simulink model "QBot2e_Path_Planning_Motion_Control"  (Simulink 8.9)
settings: Solver=ode1  StartTime=0.0  StopTime=inf  FixedStep=0.01  RelTol=1e-3  EnableMultiTasking=on
values from neighbouring files (symbols this model uses):
  px = wx    [Path_Planning_MAP.m]    (also in Process_MAP.m = coords(:, 1))
  py = wy    [Path_Planning_MAP.m]    (also in Process_MAP.m = coords(:, 2))
undefined symbols (not defined in the file or in its folder): HIL
libraries: quarc_library x8
settings Model: Creator=drmadill  LastModifiedBy=amolki  SimulationMode=external  ExtModeTrigDuration=1
settings SolverCC: PositivePriorityOrder=on
settings OptimizationCC: ExpressionDepthLimit=2147483647  LifeSpan=auto
settings DebuggingCC: SolverPrmCheckMsg=warning
settings RTWCC: SystemTargetFile=quarc_linux_pi_3.tlc  TemplateMakefile=quarc_linux_pi_3_tmf  Description=QUARC Linux Raspberry Pi 3 Target
settings STFCustomTargetCC: TargetLibSuffix=.a  TargetPreCompLibLocation=C:\PROGRA~3\QUARC\lib\2017a\LICFC8~1\release  ConcurrentExecutionCompliant=on  SystemTargetFile=quarc_linux_pi_3.tlc
settings GRTTargetCC: TargetLibSuffix=.a  TargetPreCompLibLocation=C:\PROGRA~3\QUARC\lib\2017a\LICFC8~1\release  ParMdlRefBuildCompliant=off  CompOptLevelCompliant=off  GeneratePreprocessorConditionals=Use local settings  MatFileLogging=off  CPPClassGenCompliant=off  UseToolchainInfoCompliant=off  ExtMode=on  ExtModeMexFile=quarc_comm  ExtModeMexArgs='-w -d /tmp -uri %u'
settings ConfigComp: CovSFcnEnable=off

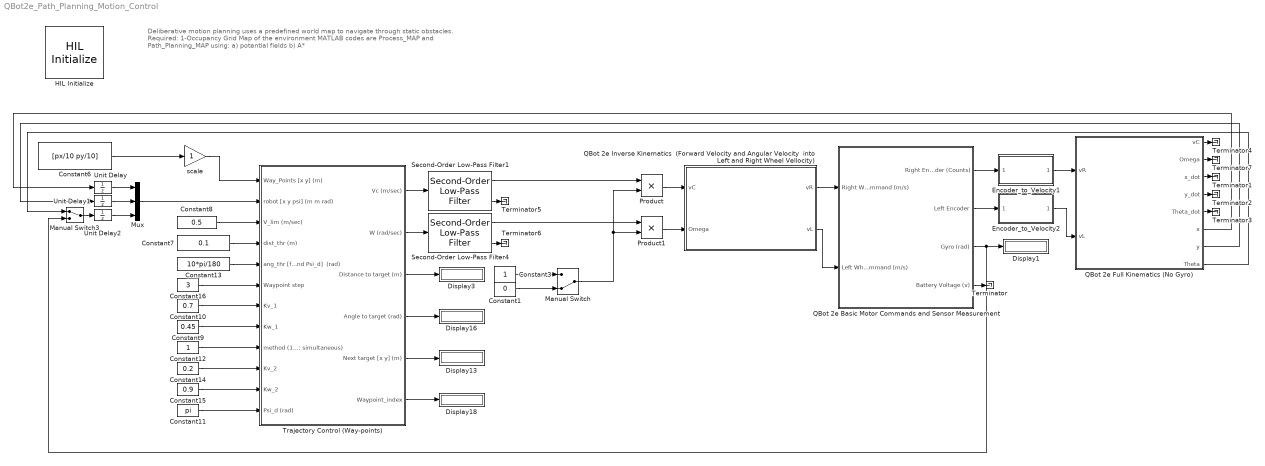
== system QBot2e_Path_Planning_Motion_Control ==
  note: Deliberative motion planning uses a predefined world map to navigate through static obstacles.
      |
      | Required:
      | 1-Occupancy Grid Map of the environment
      | MATLAB codes are Process_MAP and Path_Planning_MAP using:
      | a) potential fields
      | b) A*
  Constant1 : Constant  Value=0
  Constant10 : Constant  Value=0.7
  Constant11 : Constant  Value=pi
  Constant12 : Constant
  Constant13 : Constant  Value=10*pi/180
  Constant14 : Constant  Value=0.2
  Constant15 : Constant  Value=0.9
  Constant16 : Constant  Value=3
  Constant3 : Constant
  Constant6 : Constant  Value=[px/10 py/10]  OutDataTypeStr=double
  Constant7 : Constant  Value=0.1
  Constant8 : Constant  Value=0.5
  Constant9 : Constant  Value=0.45
  Display{1,3,13,16,18} (5 alike) : Display
  Encoder_to_Velocity1 : Subsystem
  Encoder_to_Velocity2 : Subsystem
  HIL Initialize : quarc_library/Data Acquisition/Generic/Configuration/HIL Initialize  Priority=-99  object_name=HIL-1  board_type=qbot2e  board_number=0  board_options=pwm0_en=1;pwm0_pin=12;pwm1_en=1;pwm1_pin=13;  exclusive=off  active=off  hardware_clocks=[]  clock_modes=[]  initial_clock_frequencies=[]  set_clock_params_at_start=off  set_clock_params_at_switch_in=off  set_clock_frequencies_at_start=off  set_clock_frequencies_at_switch_in=off  analog_input_channels=[0:5]  analog_input_configurations=[]  analog_input_maximums=[16.5 3.3 3.3 3.3 3.3 3.3]  analog_input_minimums=[0 0 0 0 0 0]  set_analog_input_params_at_start=off  set_analog_input_params_at_switch_in=off  analog_output_channels=[]  analog_output_maximums=[]  analog_output_minimums=[]  initial_analog_outputs=[]  final_analog_outputs=[]  watchdog_analog_outputs=[]  set_analog_output_params_at_start=off  set_analog_output_params_at_switch_in=off  set_analog_outputs_at_start=off  set_analog_outputs_at_switch_in=off  set_analog_outputs_at_terminate=off  set_analog_outputs_at_switch_out=off  set_analog_outputs_on_watchdog=off  digital_input_channels=[28:58]  digital_output_channels=[28:31]  digital_output_configuration=[]  initial_digital_outputs=[0]  final_digital_outputs=[0]  watchdog_digital_outputs=[]  set_digital_output_params_at_start=off  set_digital_output_params_at_switch_in=off  set_digital_outputs_at_start=on  set_digital_outputs_at_switch_in=off  set_digital_outputs_at_terminate=on  set_digital_outputs_at_switch_out=off  set_digital_outputs_on_watchdog=off  encoder_channels=[0:1]  quadrature=[4]  encoder_filter_frequency=[]  initial_encoder_counts=[0]  set_encoder_params_at_start=on  set_encoder_params_at_switch_in=off  set_encoder_counts_at_start=on  set_encoder_counts_at_switch_in=off  pwm_channels=[0:1]  pwm_modes=0  pwm_frequency=100e6 / 4095  pwm_configuration=[0]  pwm_alignment=[0]  pwm_polarity=[1]  pwm_leading_deadband=[]  pwm_trailing_deadband=[]  initial_pwm_outputs=[0]  final_pwm_outputs=[0]  watchdog_pwm_outputs=[]  set_pwm_params_at_start=on  set_pwm_params_at_switch_in=off  set_pwm_outputs_at_start=on  set_pwm_outputs_at_switch_in=off  set_pwm_outputs_at_terminate=on  set_pwm_outputs_at_switch_out=off  set_pwm_outputs_on_watchdog=off  other_output_channels=[2000:2001 14000 16000]  initial_other_outputs=[0 0 0 7]  final_other_outputs=[0 0 0 7]  watchdog_other_outputs=[]  set_other_outputs_at_start=on  set_other_outputs_at_switch_in=off  set_other_outputs_at_terminate=on  set_other_outputs_at_switch_out=off  set_other_outputs_on_watchdog=off
  Manual Switch : ManualSwitch  CurrentSetting=0
  Manual Switch3 : ManualSwitch
  Mux : Mux  Inputs=[1 1 1]
  Product : Product  RndMeth=Zero
  Product1 : Product  RndMeth=Zero
  QBot 2e Basic Motor Commands and Sensor Measurement : Subsystem
  QBot 2e Full Kinematics (No Gyro) : Subsystem
  QBot 2e Inverse Kinematics  (Forward Velocity and Angular Velocity  into Left and Right Wheel Vellocity) : Subsystem
  Second-Order Low-Pass Filter1 : quarc_library/Continuous/Second-Order Low-Pass Filter  params_source=Internal (dialog parameters)  input_width=30  input_zeta=1  input_init=0
  Second-Order Low-Pass Filter4 : quarc_library/Continuous/Second-Order Low-Pass Filter  params_source=Internal (dialog parameters)  input_width=60  input_zeta=1  input_init=0
  Terminator{,1..7} (8 alike) : Terminator
  Trajectory Control (Way-points) : Subsystem
  Unit Delay : UnitDelay  SampleTime=-1
  Unit Delay1 : UnitDelay  SampleTime=-1
  Unit Delay2 : UnitDelay  SampleTime=-1
  scale : Gain
  wires:
  Constant3/1 -> Manual Switch/1
  Constant1/1 -> Manual Switch/2
  QBot 2e Basic Motor Commands and Sensor Measurement/1(Right Encoder (Counts)) -> Encoder_to_Velocity1/1(Encoder)
  QBot 2e Basic Motor Commands and Sensor Measurement/2(Left Encoder) -> Encoder_to_Velocity2/1(Encoder)
  QBot 2e Basic Motor Commands and Sensor Measurement/3(Gyro (rad)) -> Display1/1, Manual Switch3/2
  QBot 2e Full Kinematics (No Gyro)/8(Theta) -> Manual Switch3/1
  Encoder_to_Velocity1/1(Velocity) -> QBot 2e Full Kinematics (No Gyro)/1(vR)
  Encoder_to_Velocity2/1(Velocity) -> QBot 2e Full Kinematics (No Gyro)/2(vL)
  Second-Order Low-Pass Filter1/1 -> Product/1
  Second-Order Low-Pass Filter4/1 -> Product1/1
  QBot 2e Inverse Kinematics  (Forward Velocity and Angular Velocity  into Left and Right Wheel Vellocity)/1(vR) -> QBot 2e Basic Motor Commands and Sensor Measurement/1(Right Wheel Command (m/s))
  QBot 2e Inverse Kinematics  (Forward Velocity and Angular Velocity  into Left and Right Wheel Vellocity)/2(vL) -> QBot 2e Basic Motor Commands and Sensor Measurement/2(Left Wheel Command (m/s))
  Product/1 -> QBot 2e Inverse Kinematics  (Forward Velocity and Angular Velocity  into Left and Right Wheel Vellocity)/1(vC)
  Product1/1 -> QBot 2e Inverse Kinematics  (Forward Velocity and Angular Velocity  into Left and Right Wheel Vellocity)/2(Omega)
  Manual Switch/1 -> Product/2, Product1/2
  QBot 2e Full Kinematics (No Gyro)/3(x_dot) -> Terminator1/1
  QBot 2e Full Kinematics (No Gyro)/4(y_dot) -> Terminator2/1
  QBot 2e Full Kinematics (No Gyro)/5(Theta_dot) -> Terminator3/1
  Constant8/1 -> Trajectory Control (Way-points)/3(V_lim (m/sec))
  Constant6/1 -> scale/1
  Constant7/1 -> Trajectory Control (Way-points)/4(dist_thr (m))
  Constant13/1 -> Trajectory Control (Way-points)/5(ang_thr [for method 1 and Psi_d]  (rad))
  Constant16/1 -> Trajectory Control (Way-points)/6(Waypoint step)
  Trajectory Control (Way-points)/3(Distance to target (m)) -> Display3/1
  Mux/1 -> Trajectory Control (Way-points)/2(robot [x y psi] (m m rad))
  Unit Delay/1 -> Mux/1
  Unit Delay1/1 -> Mux/2
  Unit Delay2/1 -> Mux/3
  Constant10/1 -> Trajectory Control (Way-points)/7(Kv_1)
  Constant9/1 -> Trajectory Control (Way-points)/8(Kw_1)
  Trajectory Control (Way-points)/4(Angle to target (rad)) -> Display16/1
  scale/1 -> Trajectory Control (Way-points)/1(Way_Points [x y] (m))
  Trajectory Control (Way-points)/1(Vc (m/sec)) -> Second-Order Low-Pass Filter1/1
  Trajectory Control (Way-points)/2(W (rad/sec)) -> Second-Order Low-Pass Filter4/1
  Manual Switch3/1 -> Unit Delay2/1
  Trajectory Control (Way-points)/5(Next target [x y] (m)) -> Display13/1
  Constant14/1 -> Trajectory Control (Way-points)/10(Kv_2)
  Constant15/1 -> Trajectory Control (Way-points)/11(Kw_2)
  Constant12/1 -> Trajectory Control (Way-points)/9("method (1: sequential, 2: simultaneous)")
  Constant11/1 -> Trajectory Control (Way-points)/12(Psi_d (rad))
  Trajectory Control (Way-points)/6(Waypoint_index) -> Display18/1
  QBot 2e Full Kinematics (No Gyro)/6(x) -> Unit Delay/1
  QBot 2e Full Kinematics (No Gyro)/7(y) -> Unit Delay1/1
  Second-Order Low-Pass Filter1/2 -> Terminator5/1
  Second-Order Low-Pass Filter4/2 -> Terminator6/1
  QBot 2e Full Kinematics (No Gyro)/1(vC) -> Terminator4/1
  QBot 2e Full Kinematics (No Gyro)/2(Omega) -> Terminator7/1
  QBot 2e Basic Motor Commands and Sensor Measurement/4(Battery Voltage (v)) -> Terminator/1

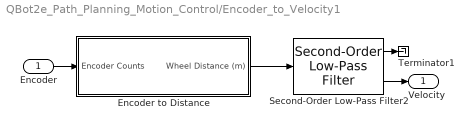
== system QBot2e_Path_Planning_Motion_Control/Encoder_to_Velocity1 ==
  Encoder : Inport
  Encoder to Distance : Subsystem
  Second-Order Low-Pass Filter2 : quarc_library/Continuous/Second-Order Low-Pass Filter  params_source=Internal (dialog parameters)  input_width=10  input_zeta=1  input_init=0
  Terminator1 : Terminator
  Velocity : Outport
  wires:
  Second-Order Low-Pass Filter2/1 -> Terminator1/1
  Encoder to Distance/1(Wheel Distance (m)) -> Second-Order Low-Pass Filter2/1
  Encoder/1 -> Encoder to Distance/1(Encoder Counts)
  Second-Order Low-Pass Filter2/2 -> Velocity/1

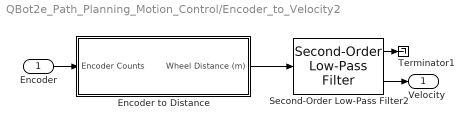
== system QBot2e_Path_Planning_Motion_Control/Encoder_to_Velocity2 ==
  Encoder : Inport
  Encoder to Distance : Subsystem
  Second-Order Low-Pass Filter2 : quarc_library/Continuous/Second-Order Low-Pass Filter  params_source=Internal (dialog parameters)  input_width=10  input_zeta=1  input_init=0
  Terminator1 : Terminator
  Velocity : Outport
  wires:
  Second-Order Low-Pass Filter2/2 -> Velocity/1
  Encoder/1 -> Encoder to Distance/1(Encoder Counts)
  Encoder to Distance/1(Wheel Distance (m)) -> Second-Order Low-Pass Filter2/1
  Second-Order Low-Pass Filter2/1 -> Terminator1/1

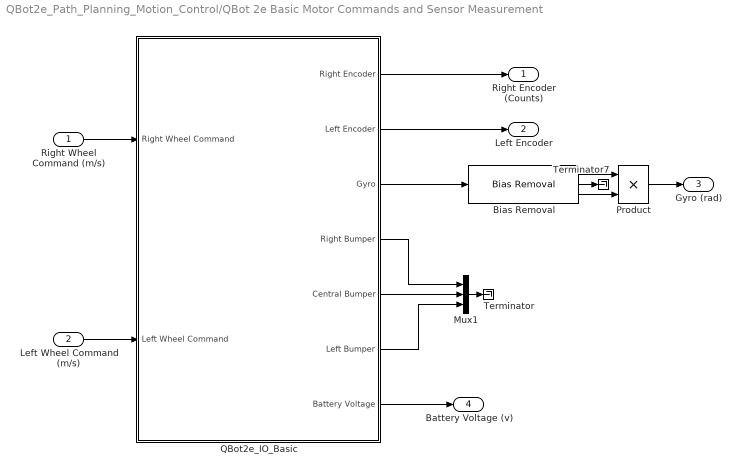
== system QBot2e_Path_Planning_Motion_Control/QBot 2e Basic Motor Commands and Sensor Measurement ==
  Right Wheel Command (m/s) : Inport
  Left Wheel Command (m/s) : Inport  Port=2
  Bias Removal : quarc_library/Discrete/Bias Removal  start_time=3  end_time=4  switch_id=0  sample_time=qc_get_step_size
      settings: SourceProductName=QUARC Targets
  Mux1 : Mux  Inputs=3
  Product : Product  RndMeth=Zero
  QBot2e_IO_Basic : Subsystem
  Terminator : Terminator
  Terminator7 : Terminator
  Right Encoder (Counts) : Outport
  Left Encoder : Outport  Port=2
  Gyro (rad) : Outport  Port=3
  Battery Voltage (v) : Outport  Port=4
  wires:
  QBot2e_IO_Basic/4(Right Bumper) -> Mux1/1
  QBot2e_IO_Basic/5(Central Bumper) -> Mux1/2
  QBot2e_IO_Basic/6(Left Bumper) -> Mux1/3
  Right Wheel Command (m/s)/1 -> QBot2e_IO_Basic/1(Right Wheel Command)
  Left Wheel Command (m/s)/1 -> QBot2e_IO_Basic/2(Left Wheel Command)
  QBot2e_IO_Basic/1(Right Encoder) -> Right Encoder (Counts)/1
  QBot2e_IO_Basic/2(Left Encoder) -> Left Encoder/1
  QBot2e_IO_Basic/7(Battery Voltage) -> Battery Voltage (v)/1
  Bias Removal/2 -> Terminator7/1
  Bias Removal/1 -> Product/1
  Bias Removal/3 -> Product/2
  Product/1 -> Gyro (rad)/1
  QBot2e_IO_Basic/3(Gyro) -> Bias Removal/1
  Mux1/1 -> Terminator/1

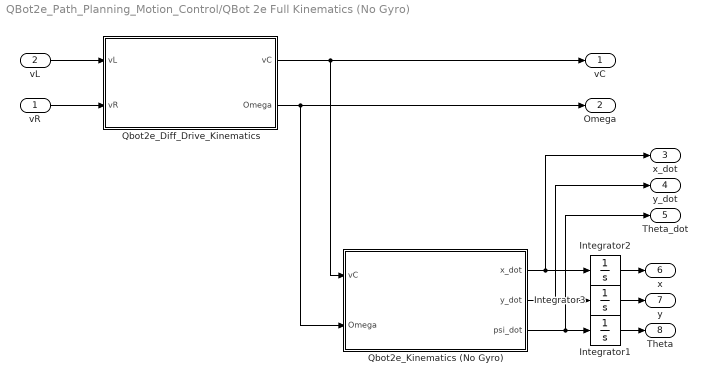
== system QBot2e_Path_Planning_Motion_Control/QBot 2e Full Kinematics (No Gyro) ==
  vR : Inport
  vL : Inport  Port=2
  Integrator1 : Integrator
  Integrator2 : Integrator
  Integrator3 : Integrator
  Qbot2e_Diff_Drive_Kinematics : Subsystem
  Qbot2e_Kinematics (No Gyro) : Subsystem
  vC : Outport
  Omega : Outport  Port=2
  x_dot : Outport  Port=3
  y_dot : Outport  Port=4
  Theta_dot : Outport  Port=5
  x : Outport  Port=6
  y : Outport  Port=7
  Theta : Outport  Port=8
  wires:
  Integrator1/1 -> Theta/1
  Qbot2e_Kinematics (No Gyro)/3(psi_dot) -> Theta_dot/1, Integrator1/1
  Qbot2e_Kinematics (No Gyro)/1(x_dot) -> x_dot/1, Integrator2/1
  Qbot2e_Kinematics (No Gyro)/2(y_dot) -> y_dot/1, Integrator3/1
  Qbot2e_Diff_Drive_Kinematics/1(vC) -> Qbot2e_Kinematics (No Gyro)/1(vC), vC/1
  vL/1 -> Qbot2e_Diff_Drive_Kinematics/1(vL)
  vR/1 -> Qbot2e_Diff_Drive_Kinematics/2(vR)
  Integrator2/1 -> x/1
  Integrator3/1 -> y/1
  Qbot2e_Diff_Drive_Kinematics/2(Omega) -> Qbot2e_Kinematics (No Gyro)/2(Omega), Omega/1

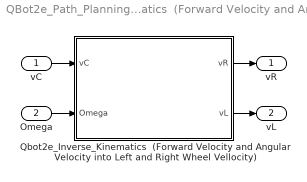
== system QBot2e_Path_Planning_Motion_Control/QBot 2e Inverse Kinematics  (Forward Velocity and Angular Velocity  into Left and Right Wheel Vellocity) ==
  vC : Inport
  Omega : Inport  Port=2
  Qbot2e_Inverse_Kinematics  (Forward Velocity and Angular Velocity into Left and Right Wheel Vellocity) : MATLAB Function  TreatAsAtomicUnit=on
  vR : Outport
  vL : Outport  Port=2
  wires:
  Qbot2e_Inverse_Kinematics  (Forward Velocity and Angular Velocity into Left and Right Wheel Vellocity)/2(vL) -> vL/1
  Omega/1 -> Qbot2e_Inverse_Kinematics  (Forward Velocity and Angular Velocity into Left and Right Wheel Vellocity)/2(Omega)
  Qbot2e_Inverse_Kinematics  (Forward Velocity and Angular Velocity into Left and Right Wheel Vellocity)/1(vR) -> vR/1
  vC/1 -> Qbot2e_Inverse_Kinematics  (Forward Velocity and Angular Velocity into Left and Right Wheel Vellocity)/1(vC)

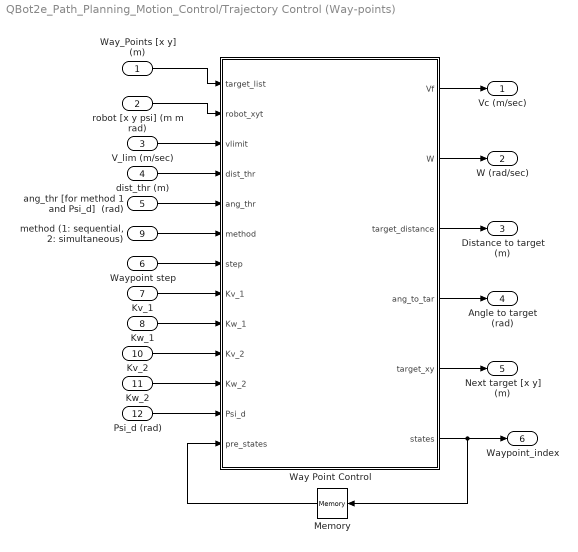
== system QBot2e_Path_Planning_Motion_Control/Trajectory Control (Way-points) ==
  Way_Points [x y] (m) : Inport
  robot [x y psi] (m m rad) : Inport  Port=2
  V_lim (m/sec) : Inport  Port=3
  dist_thr (m) : Inport  Port=4
  ang_thr [for method 1 and Psi_d]  (rad) : Inport  Port=5
  Waypoint step : Inport  Port=6
  Kv_1 : Inport  Port=7
  Kw_1 : Inport  Port=8
  "method (1: sequential, 2: simultaneous)" : Inport  Port=9
  Kv_2 : Inport  Port=10
  Kw_2 : Inport  Port=11
  Psi_d (rad) : Inport  Port=12
  Memory : Memory  X0=[0]
  Way Point Control : MATLAB Function  TreatAsAtomicUnit=on
  Vc (m/sec) : Outport
  W (rad/sec) : Outport  Port=2
  Distance to target (m) : Outport  Port=3
  Angle to target (rad) : Outport  Port=4
  Next target [x y] (m) : Outport  Port=5
  Waypoint_index : Outport  Port=6
  wires:
  Memory/1 -> Way Point Control/13(pre_states)
  Way Point Control/6(states) -> Memory/1, Waypoint_index/1
  Way_Points [x y] (m)/1 -> Way Point Control/1(target_list)
  Way Point Control/1(Vf) -> Vc (m/sec)/1
  robot [x y psi] (m m rad)/1 -> Way Point Control/2(robot_xyt)
  V_lim (m/sec)/1 -> Way Point Control/3(vlimit)
  Way Point Control/2(W) -> W (rad/sec)/1
  dist_thr (m)/1 -> Way Point Control/4(dist_thr)
  Way Point Control/3(target_distance) -> Distance to target (m)/1
  ang_thr [for method 1 and Psi_d]  (rad)/1 -> Way Point Control/5(ang_thr)
  Way Point Control/4(ang_to_tar) -> Angle to target (rad)/1
  Waypoint step/1 -> Way Point Control/7(step)
  Kv_1/1 -> Way Point Control/8(Kv_1)
  Way Point Control/5(target_xy) -> Next target [x y] (m)/1
  Kw_1/1 -> Way Point Control/9(Kw_1)
  "method (1: sequential, 2: simultaneous)"/1 -> Way Point Control/6(method)
  Kv_2/1 -> Way Point Control/10(Kv_2)
  Kw_2/1 -> Way Point Control/11(Kw_2)
  Psi_d (rad)/1 -> Way Point Control/12(Psi_d)

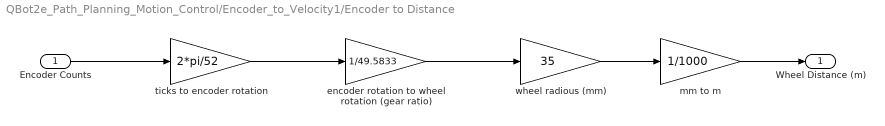
== system QBot2e_Path_Planning_Motion_Control/Encoder_to_Velocity1/Encoder to Distance ==
  Encoder Counts : Inport
  " encoder rotation to wheel rotation (gear ratio)" : Gain  Gain=1/49.5833
  mm to m : Gain  Gain=1/1000
  ticks to encoder rotation : Gain  Gain=2*pi/52
  wheel radious (mm) : Gain  Gain=35
  Wheel Distance (m) : Outport
  wires:
  Encoder Counts/1 -> ticks to encoder rotation/1
  ticks to encoder rotation/1 -> " encoder rotation to wheel rotation (gear ratio)"/1
  " encoder rotation to wheel rotation (gear ratio)"/1 -> wheel radious (mm)/1
  wheel radious (mm)/1 -> mm to m/1
  mm to m/1 -> Wheel Distance (m)/1

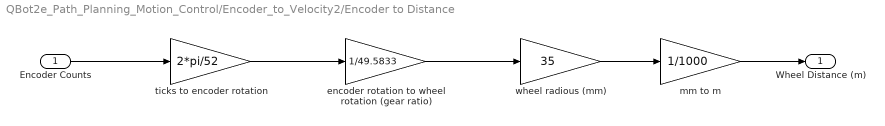
== system QBot2e_Path_Planning_Motion_Control/Encoder_to_Velocity2/Encoder to Distance ==
  Encoder Counts : Inport
  " encoder rotation to wheel rotation (gear ratio)" : Gain  Gain=1/49.5833
  mm to m : Gain  Gain=1/1000
  ticks to encoder rotation : Gain  Gain=2*pi/52
  wheel radious (mm) : Gain  Gain=35
  Wheel Distance (m) : Outport
  wires:
  mm to m/1 -> Wheel Distance (m)/1
  wheel radious (mm)/1 -> mm to m/1
  " encoder rotation to wheel rotation (gear ratio)"/1 -> wheel radious (mm)/1
  ticks to encoder rotation/1 -> " encoder rotation to wheel rotation (gear ratio)"/1
  Encoder Counts/1 -> ticks to encoder rotation/1

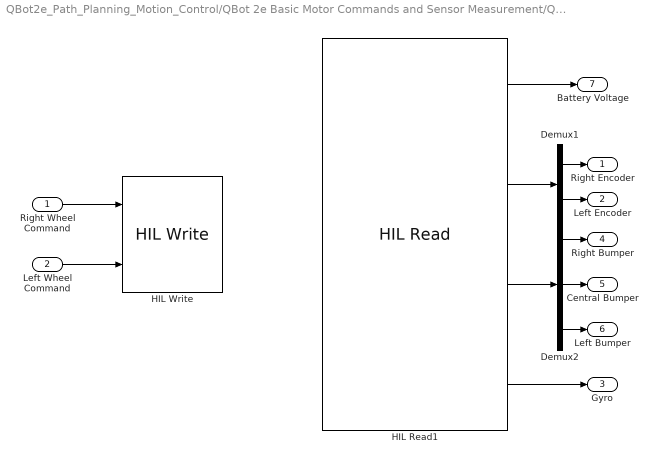
== system QBot2e_Path_Planning_Motion_Control/QBot 2e Basic Motor Commands and Sensor Measurement/QBot2e_IO_Basic ==
  Right Wheel Command : Inport
  Left Wheel Command : Inport  Port=2
  Demux1 : Demux  Outputs=2
  Demux2 : Demux  Outputs=3
  HIL Read1 : quarc_library/Data Acquisition/Generic/Immediate I//O/HIL Read  object_name=HIL-1  analog_channels=[0]  encoder_channels=[0:1]  digital_channels=[28:30]  other_channels=[1002]  sample_time=qc_get_step_size  active=on  vector_output=on  data_type_mode=Inherit via back propagation  encoder_data_type=double  digital_data_type=boolean
  HIL Write : quarc_library/Data Acquisition/Generic/Immediate I//O/HIL Write  object_name=HIL-1  analog_channels=[]  pwm_channels=[]  digital_channels=[]  other_channels=[2000:2001]  sample_time=-1  active=on  vector_input=off
  Right Encoder : Outport
  Left Encoder : Outport  Port=2
  Gyro : Outport  Port=3
  Right Bumper : Outport  Port=4
  Central Bumper : Outport  Port=5
  Left Bumper : Outport  Port=6
  Battery Voltage : Outport  Port=7
  wires:
  HIL Read1/1 -> Battery Voltage/1
  HIL Read1/3 -> Demux2/1
  HIL Read1/4 -> Gyro/1
  Demux1/1 -> Right Encoder/1
  Demux1/2 -> Left Encoder/1
  Right Wheel Command/1 -> HIL Write/1
  Left Wheel Command/1 -> HIL Write/2
  HIL Read1/2 -> Demux1/1
  Demux2/1 -> Right Bumper/1
  Demux2/2 -> Central Bumper/1
  Demux2/3 -> Left Bumper/1

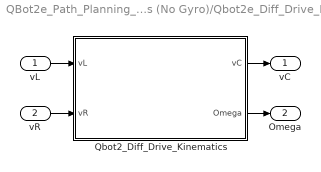
== system QBot2e_Path_Planning_Motion_Control/QBot 2e Full Kinematics (No Gyro)/Qbot2e_Diff_Drive_Kinematics ==
  vL : Inport
  vR : Inport  Port=2
  Qbot2_Diff_Drive_Kinematics : MATLAB Function  TreatAsAtomicUnit=on
  vC : Outport
  Omega : Outport  Port=2
  wires:
  vL/1 -> Qbot2_Diff_Drive_Kinematics/1(vL)
  Qbot2_Diff_Drive_Kinematics/1(vC) -> vC/1
  vR/1 -> Qbot2_Diff_Drive_Kinematics/2(vR)
  Qbot2_Diff_Drive_Kinematics/2(Omega) -> Omega/1

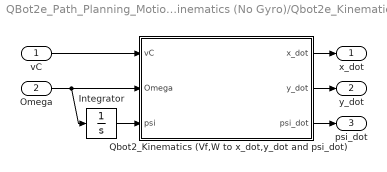
== system QBot2e_Path_Planning_Motion_Control/QBot 2e Full Kinematics (No Gyro)/Qbot2e_Kinematics (No Gyro) ==
  vC : Inport
  Omega : Inport  Port=2
  Integrator : Integrator
  Qbot2_Kinematics (Vf,W to x_dot,y_dot and psi_dot) : MATLAB Function  TreatAsAtomicUnit=on
  x_dot : Outport
  y_dot : Outport  Port=2
  psi_dot : Outport  Port=3
  wires:
  Qbot2_Kinematics (Vf,W to x_dot,y_dot and psi_dot)/3(psi_dot) -> psi_dot/1
  Integrator/1 -> Qbot2_Kinematics (Vf,W to x_dot,y_dot and psi_dot)/3(psi)
  vC/1 -> Qbot2_Kinematics (Vf,W to x_dot,y_dot and psi_dot)/1(vC)
  Qbot2_Kinematics (Vf,W to x_dot,y_dot and psi_dot)/1(x_dot) -> x_dot/1
  Omega/1 -> Integrator/1, Qbot2_Kinematics (Vf,W to x_dot,y_dot and psi_dot)/2(Omega)
  Qbot2_Kinematics (Vf,W to x_dot,y_dot and psi_dot)/2(y_dot) -> y_dot/1

== matlab function QBot 2e Full Kinematics (No Gyro)/Qbot2e_Diff_Drive_Kinematics/Qbot2_Diff_Drive_Kinematics ==
  data: vL input double; vC output double; vR input double; Omega output double
function [vC,Omega] = fcn(vL,vR)
%#codegen

d= 0.235;

vC=0.5*(vL+vR);
Omega=(1/d)*(vR-vL);

== matlab function QBot 2e Full Kinematics (No Gyro)/Qbot2e_Kinematics (No Gyro)/Qbot2_Kinematics (Vf,W to x_dot,y_dot and psi_dot) ==
  data: vC input double; x_dot output double; Omega input double; y_dot output double; psi input double; psi_dot output double
function [x_dot,y_dot,psi_dot] = fcn(vC,Omega,psi)
%#codegen


x_dot=cos(psi)*vC;
y_dot=sin(psi)*vC;
psi_dot= Omega;

== matlab function Trajectory Control (Way-points)/Way Point Control ==
  data: target_list input double; robot_xyt input double; vlimit input double; dist_thr input double; ang_thr input double; method input double; step input double; Kv_1 input double; Kw_1 input double; Kv_2 input double; Kw_2 input double; Psi_d input double; Vf output double; W output double; target_distance output double; ang_to_tar output double; target_xy output double; states output double; pre_states input double
function [Vf, W, target_distance, ang_to_tar, target_xy, states] = ...
    WaypointControl(target_list, robot_xyt, vlimit, ...
    dist_thr, ang_thr, method, step, Kv_1, Kw_1, Kv_2, Kw_2, Psi_d, pre_states)

% Initialize output variables

 Vf=0;
 W=0;
 finished_path_flag=0; 
 
 persistent Vf_1 end_flag;
 
 if isempty(Vf_1)
     Vf_1=0;
 end
 if isempty(end_flag)
    end_flag = 0;
 end
states = pre_states;



rx = robot_xyt(1);
ry = robot_xyt(2);
rtheta = check_angle(robot_xyt(3));
target_xy = [rx ry];
[n xy] = size(target_list);
if n==2 && xy==1
    target_xy = [target_list(1,1) target_list(2,1)];
    n = 1;
else
    for i=1:n
        if states(1) == i
            for j=1:xy
                target_xy(j) = target_list(i, j);
            end
        end
    end
end

tx = target_xy(1);
ty = target_xy(2);
target_distance = find_dist(rx, ry, tx, ty);
ang_to_tar= find_theta(rx, ry, rtheta, tx, ty);

if ((states(1) == n) && (target_distance <= dist_thr))  %|| states(1) == -1
% %        states(1) = -1;
       % right_vel = int16(0);
       % left_vel = int16(0);
%  %       target_distance = 0;
        Vf=0;
        W=0;
        
       if (end_flag == 1) && (target_distance <= dist_thr) % after all waypoints, psi will be adjusted to psi_d 
            [Vf, W] = ClosedLoop_Sequential(0, check_angle(check_angle(Psi_d)-check_angle(rtheta)), vlimit, ang_thr, dist_thr, Kv_1, Kw_1, Vf_1); 
             Vf_1=Vf;
       end
        
   
else
    
    if (target_distance <= dist_thr) && (end_flag==0)
            states(1) = pre_states(1) + step;%1;
      if( pre_states(1)>0 )      
         while (abs((target_list(states(1),1))-(target_list(pre_states(1),1)))<2*dist_thr) && (abs((target_list(states(1),2))-(target_list(pre_states(1),2)))<2*dist_thr)
             if (states(1)<=(n-step))
                 states(1) = states(1) + step;%1;
             else
                 states(1)=n;
             end
         end
      else
          states(1)=states(1)+step;
      end
         if states(1) >= n 
            states(1) = n;
            end_flag=1;
         end
        
               
  %  elseif (end_flag == 1) && (target_distance <= dist_thr) % after all waypoints, psi will be adjusted to psi_d 
  %          [Vf, W] = ClosedLoop_Sequential(0, check_angle(check_angle(Psi_d)-check_angle(rtheta)), vlimit, ang_thr, dist_thr, Kv_1, Kw_1, Vf_1); 
  %           Vf_1=Vf;
    else
        
        
            if method == 2
                [Vf, W] = ClosedLoop_Both(target_distance,  ang_to_tar, vlimit, Kv_2, Kw_2);    
            else
    %            [right_vel, left_vel] = rotate_and_go(ang_to_tar, vlimit, ang_thr);
                [Vf, W] = ClosedLoop_Sequential(target_distance,  ang_to_tar, vlimit, ang_thr, dist_thr, Kv_1, Kw_1, Vf_1); 
                Vf_1=Vf;
            end
                 
    end
end


return;

%--------------------------------------------------------------------------
function [y] = check_angle(x)
y = x;
if x > pi
    y = x - 2*pi;
elseif x < -pi
    y = x + 2*pi;
end
return;
% -------------------------------------------------------------------------
function dist = find_dist(rx, ry, tx, ty)
dist = sqrt((rx-tx)^2 + (ry-ty)^2);
return;
% -------------------------------------------------------------------------
function [theta]= find_theta(rx, ry, rtheta, tx, ty)

X = tx - rx;
Y = ty - ry;
theta = atan2(Y, X);
theta = check_angle(check_angle(theta)-check_angle(rtheta));

return;
% -------------------------------------------------------------------------

function [Vf, W] = ClosedLoop_Both(dist, theta, vlimit, Kv,Kw)

d = 0.23;
vmax = vlimit;
wmax = (2*vmax);
W = Kw*theta;

%if abs(theta)<pi
Vf = Kv*dist;
%else
%    Vf=0;
%end

w_sign = sign(W);
if abs(W) > wmax
    W = w_sign*wmax;
end
if abs(Vf)> vlimit
    Vf = abs(Vf)*vlimit;
end

return;

function [Vf, W] = ClosedLoop_Sequential(dist, theta, vlimit, ang_thr, dist_thr, Kv, Kw, Vf_1)

d = 0.23;
vmax = vlimit;
wmax = (2*vmax);

if (((abs(theta) > ang_thr))  && (Vf_1<0.01)) || (abs(theta) > 5*ang_thr) % once rotated, then moves. once started moving, it won't turn unless the heading is too off target or have reached the previous target.
        W=Kw*theta;
        Vf=0;
        if abs(W)> wmax
            W=sign(theta)*wmax;
        end
else
        Vf=Kv*dist;
       
        if abs(Vf)>vlimit
            Vf=sign(Vf)*vlimit;
        end
       % if (abs(theta) > 2*ang_thr)
       %   W=Kw*theta;
       %   Vf=0.4*Vf;
       % else
       W=0;
       % end
       % if abs(W)> wmax
       %     W=sign(theta)*wmax;
       % end
        
end

return;

%{
function [vr, vl] = solve_inv_kin(dist, theta, vlimit, delta_t)

d = 0.23;
vmax = vlimit(2);
wmax = (2*vmax)/d;
w = theta/delta_t;
w_sign = sign(w);
if abs(w) > wmax
    w = w_sign*wmax;
    vr = int16(round((d*w)/2));
    vl = int16(-vr);
else
    v = dist/delta_t;
    vr_tmp = (2*v + d*w)/2;
    vl_tmp = 2*v - vr_tmp;
    
    max_of_vrvl = abs(max(vr_tmp, vl_tmp));
    if max_of_vrvl > vmax
        vr_tmp = (vr_tmp/max_of_vrvl)*vmax;
        vl_tmp = (vl_tmp/max_of_vrvl)*vmax;
    end
    vr = int16(vr_tmp);
    vl = int16(vl_tmp);

end


return;
%}

%{
% -------------------------------------------------------------------------
function [vr, vl] = rotate_and_go(theta, vlimit, ang_thr)

if abs(theta) > ang_thr
    if theta >= 0
        vr = int16(vlimit(1));
        vl = int16(-vlimit(1));
    else
        vr = int16(-vlimit(1));
        vl = int16(vlimit(1));
    end
else
        vr = int16(vlimit(2));
        vl = int16(vlimit(2));
end

return;
% -------------------------------------------------------------------------
%}

== matlab function QBot 2e Inverse Kinematics (Forward Velocity and Angular Velocity into Left and Right Wheel Vellocity)/Qbot2e_Inverse_Kinematics (Forward Velocity and Angular Velocity into Left and Right Wheel Vellocity) ==
  data: vR output double; vL output double; vC input double; Omega input double
function [vR,vL] = fcn(vC , Omega)
%#codegen

d=0.235; 
% Eqn Based on the eqn 4.52 (W is the angular velocity)

vR = vC + Omega*d/2;
vL= vC - Omega*d/2;
